simulink model "ControlTest"  (R2016b)
settings: Solver=VariableStepAuto  StartTime=0.0  StopTime=300  MaxStep=0.05  RelTol=1e-3
values from neighbouring files (symbols this model uses):
  X0 = P.x0    [gps.m]
undefined symbols (not defined in the file or in its folder): A, B, C, D, deltaChi, drawplane, GetPosition, P
libraries: simulink x9
settings Model: Creator=CFRPG  LastModifiedBy=CFRPG
settings SolverCC: ZeroCrossAlgorithm=Adaptive

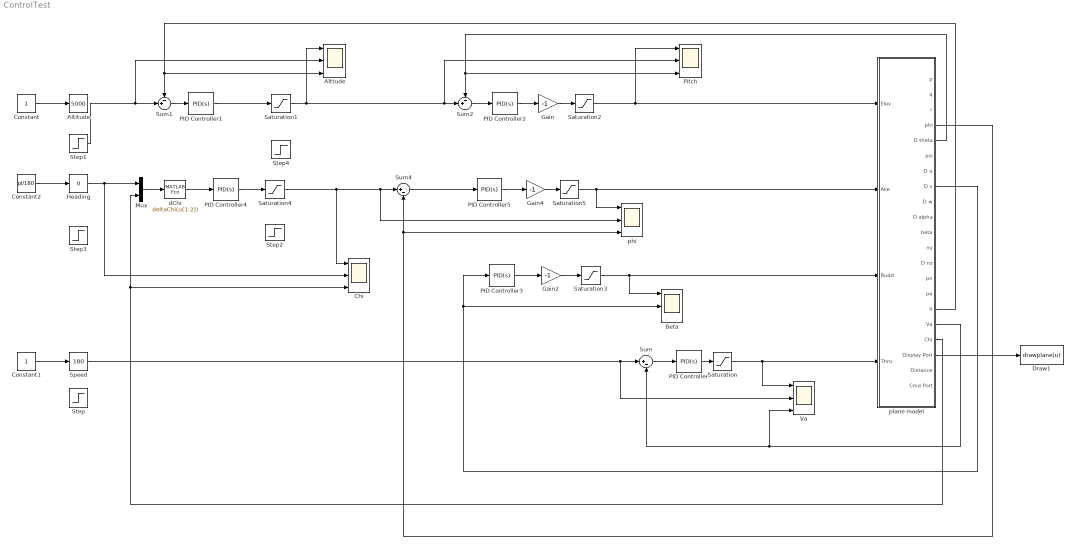
== system ControlTest ==
  Altitude : simulink/Math Operations/Slider Gain  low=0  gain=5000  high=8000
  Alttude : Scope  NumInputPorts=3
  Beta : Scope  NumInputPorts=3
  Chi : Scope  NumInputPorts=3
  Constant : Constant
  Constant1 : Constant
  Constant2 : Constant  Value=pi/180
  Draw1 : MATLABFcn  MATLABFcn=drawplane(u)  OutputDimensions=0
  Gain : Gain  Gain=-1
  Gain2 : Gain  Gain=-1
  Gain4 : Gain  Gain=-1
  Heading : simulink/Math Operations/Slider Gain  low=0  gain=0  high=360
  Mux : Mux  Inputs=2
  PID Controller : simulink/Continuous/PID Controller  Controller=PID  TimeDomain=Continuous-time  SampleTime=-1  IntegratorMethod=Forward Euler  FilterMethod=Forward Euler  Form=Parallel  UseFilter=on  ControllerParametersSource=internal  P=1.6  I=0.001  D=0.01  N=100  InitialConditionSource=internal  InitialConditionForIntegrator=0  InitialConditionForFilter=0  ExternalReset=none  LimitOutput=off  UpperSaturationLimit=inf  LowerSaturationLimit=-inf  LinearizeAsGain=on  AntiWindupMode=none  Kb=1  TrackingMode=off  Kt=1  PParamMin=[]  PParamMax=[]  IParamMin=[]  IParamMax=[]  DParamMin=[]  DParamMax=[]  NParamMin=[]  NParamMax=[]  KbParamMin=[]  KbParamMax=[]  KtParamMin=[]  KtParamMax=[]  POutMin=[]  POutMax=[]  IOutMin=[]  IOutMax=[]  DOutMin=[]  DOutMax=[]  NOutMin=[]  NOutMax=[]  KbOutMin=[]  KbOutMax=[]  KtOutMin=[]  KtOutMax=[]  IntegratorOutMin=[]  IntegratorOutMax=[]  FilterOutMin=[]  FilterOutMax=[]  SumOutMin=[]  SumOutMax=[]  SumI1OutMin=[]  SumI1OutMax=[]  SumI2OutMin=[]  SumI2OutMax=[]  SumI3OutMin=[]  SumI3OutMax=[]  SumDOutMin=[]  SumDOutMax=[]  SaturationOutMin=[]  SaturationOutMax=[]  IntegratorContinuousStateAttributes=''  IntegratorStateMustResolveToSignalObject=off  IntegratorRTWStateStorageClass=Auto  FilterContinuousStateAttributes=''  FilterStateMustResolveToSignalObject=off  FilterRTWStateStorageClass=Auto  DifferentiatorICPrevScaledInput=0  DifferentiatorOutMin=[]  DifferentiatorOutMax=[]
  PID Controller1 : simulink/Continuous/PID Controller  Controller=PID  TimeDomain=Continuous-time  SampleTime=-1  IntegratorMethod=Forward Euler  FilterMethod=Forward Euler  Form=Parallel  UseFilter=on  ControllerParametersSource=internal  P=0.02  I=0.0001  D=0.03  N=100  InitialConditionSource=internal  InitialConditionForIntegrator=0  InitialConditionForFilter=0  ExternalReset=none  LimitOutput=off  UpperSaturationLimit=inf  LowerSaturationLimit=-inf  LinearizeAsGain=on  AntiWindupMode=none  Kb=1  TrackingMode=off  Kt=1  PParamMin=[]  PParamMax=[]  IParamMin=[]  IParamMax=[]  DParamMin=[]  DParamMax=[]  NParamMin=[]  NParamMax=[]  KbParamMin=[]  KbParamMax=[]  KtParamMin=[]  KtParamMax=[]  POutMin=[]  POutMax=[]  IOutMin=[]  IOutMax=[]  DOutMin=[]  DOutMax=[]  NOutMin=[]  NOutMax=[]  KbOutMin=[]  KbOutMax=[]  KtOutMin=[]  KtOutMax=[]  IntegratorOutMin=[]  IntegratorOutMax=[]  FilterOutMin=[]  FilterOutMax=[]  SumOutMin=[]  SumOutMax=[]  SumI1OutMin=[]  SumI1OutMax=[]  SumI2OutMin=[]  SumI2OutMax=[]  SumI3OutMin=[]  SumI3OutMax=[]  SumDOutMin=[]  SumDOutMax=[]  SaturationOutMin=[]  SaturationOutMax=[]  IntegratorContinuousStateAttributes=''  IntegratorStateMustResolveToSignalObject=off  IntegratorRTWStateStorageClass=Auto  FilterContinuousStateAttributes=''  FilterStateMustResolveToSignalObject=off  FilterRTWStateStorageClass=Auto  DifferentiatorICPrevScaledInput=0  DifferentiatorOutMin=[]  DifferentiatorOutMax=[]
  PID Controller2 : simulink/Continuous/PID Controller  Controller=PID  TimeDomain=Continuous-time  SampleTime=-1  IntegratorMethod=Forward Euler  FilterMethod=Forward Euler  Form=Parallel  UseFilter=on  ControllerParametersSource=internal  P=2  I=0.1  D=0.4  N=100  InitialConditionSource=internal  InitialConditionForIntegrator=0  InitialConditionForFilter=0  ExternalReset=none  LimitOutput=off  UpperSaturationLimit=inf  LowerSaturationLimit=-inf  LinearizeAsGain=on  AntiWindupMode=none  Kb=1  TrackingMode=off  Kt=1  PParamMin=[]  PParamMax=[]  IParamMin=[]  IParamMax=[]  DParamMin=[]  DParamMax=[]  NParamMin=[]  NParamMax=[]  KbParamMin=[]  KbParamMax=[]  KtParamMin=[]  KtParamMax=[]  POutMin=[]  POutMax=[]  IOutMin=[]  IOutMax=[]  DOutMin=[]  DOutMax=[]  NOutMin=[]  NOutMax=[]  KbOutMin=[]  KbOutMax=[]  KtOutMin=[]  KtOutMax=[]  IntegratorOutMin=[]  IntegratorOutMax=[]  FilterOutMin=[]  FilterOutMax=[]  SumOutMin=[]  SumOutMax=[]  SumI1OutMin=[]  SumI1OutMax=[]  SumI2OutMin=[]  SumI2OutMax=[]  SumI3OutMin=[]  SumI3OutMax=[]  SumDOutMin=[]  SumDOutMax=[]  SaturationOutMin=[]  SaturationOutMax=[]  IntegratorContinuousStateAttributes=''  IntegratorStateMustResolveToSignalObject=off  IntegratorRTWStateStorageClass=Auto  FilterContinuousStateAttributes=''  FilterStateMustResolveToSignalObject=off  FilterRTWStateStorageClass=Auto  DifferentiatorICPrevScaledInput=0  DifferentiatorOutMin=[]  DifferentiatorOutMax=[]
  PID Controller3 : simulink/Continuous/PID Controller  Controller=PID  TimeDomain=Continuous-time  SampleTime=-1  IntegratorMethod=Forward Euler  FilterMethod=Forward Euler  Form=Parallel  UseFilter=on  ControllerParametersSource=internal  P=0.01  I=0  D=0.01  N=100  InitialConditionSource=internal  InitialConditionForIntegrator=0  InitialConditionForFilter=0  ExternalReset=none  LimitOutput=off  UpperSaturationLimit=inf  LowerSaturationLimit=-inf  LinearizeAsGain=on  AntiWindupMode=none  Kb=1  TrackingMode=off  Kt=1  PParamMin=[]  PParamMax=[]  IParamMin=[]  IParamMax=[]  DParamMin=[]  DParamMax=[]  NParamMin=[]  NParamMax=[]  KbParamMin=[]  KbParamMax=[]  KtParamMin=[]  KtParamMax=[]  POutMin=[]  POutMax=[]  IOutMin=[]  IOutMax=[]  DOutMin=[]  DOutMax=[]  NOutMin=[]  NOutMax=[]  KbOutMin=[]  KbOutMax=[]  KtOutMin=[]  KtOutMax=[]  IntegratorOutMin=[]  IntegratorOutMax=[]  FilterOutMin=[]  FilterOutMax=[]  SumOutMin=[]  SumOutMax=[]  SumI1OutMin=[]  SumI1OutMax=[]  SumI2OutMin=[]  SumI2OutMax=[]  SumI3OutMin=[]  SumI3OutMax=[]  SumDOutMin=[]  SumDOutMax=[]  SaturationOutMin=[]  SaturationOutMax=[]  IntegratorContinuousStateAttributes=''  IntegratorStateMustResolveToSignalObject=off  IntegratorRTWStateStorageClass=Auto  FilterContinuousStateAttributes=''  FilterStateMustResolveToSignalObject=off  FilterRTWStateStorageClass=Auto  DifferentiatorICPrevScaledInput=0  DifferentiatorOutMin=[]  DifferentiatorOutMax=[]
  PID Controller4 : simulink/Continuous/PID Controller  Controller=PID  TimeDomain=Continuous-time  SampleTime=-1  IntegratorMethod=Forward Euler  FilterMethod=Forward Euler  Form=Parallel  UseFilter=on  ControllerParametersSource=internal  P=1.5  I=0  D=1.2  N=100  InitialConditionSource=internal  InitialConditionForIntegrator=0  InitialConditionForFilter=0  ExternalReset=none  LimitOutput=off  UpperSaturationLimit=inf  LowerSaturationLimit=-inf  LinearizeAsGain=on  AntiWindupMode=none  Kb=1  TrackingMode=off  Kt=1  PParamMin=[]  PParamMax=[]  IParamMin=[]  IParamMax=[]  DParamMin=[]  DParamMax=[]  NParamMin=[]  NParamMax=[]  KbParamMin=[]  KbParamMax=[]  KtParamMin=[]  KtParamMax=[]  POutMin=[]  POutMax=[]  IOutMin=[]  IOutMax=[]  DOutMin=[]  DOutMax=[]  NOutMin=[]  NOutMax=[]  KbOutMin=[]  KbOutMax=[]  KtOutMin=[]  KtOutMax=[]  IntegratorOutMin=[]  IntegratorOutMax=[]  FilterOutMin=[]  FilterOutMax=[]  SumOutMin=[]  SumOutMax=[]  SumI1OutMin=[]  SumI1OutMax=[]  SumI2OutMin=[]  SumI2OutMax=[]  SumI3OutMin=[]  SumI3OutMax=[]  SumDOutMin=[]  SumDOutMax=[]  SaturationOutMin=[]  SaturationOutMax=[]  IntegratorContinuousStateAttributes=''  IntegratorStateMustResolveToSignalObject=off  IntegratorRTWStateStorageClass=Auto  FilterContinuousStateAttributes=''  FilterStateMustResolveToSignalObject=off  FilterRTWStateStorageClass=Auto  DifferentiatorICPrevScaledInput=0  DifferentiatorOutMin=[]  DifferentiatorOutMax=[]
  PID Controller5 : simulink/Continuous/PID Controller  Controller=PID  TimeDomain=Continuous-time  SampleTime=-1  IntegratorMethod=Forward Euler  FilterMethod=Forward Euler  Form=Parallel  UseFilter=on  ControllerParametersSource=internal  P=2  I=0  D=0.1  N=100  InitialConditionSource=internal  InitialConditionForIntegrator=0  InitialConditionForFilter=0  ExternalReset=none  LimitOutput=off  UpperSaturationLimit=inf  LowerSaturationLimit=-inf  LinearizeAsGain=on  AntiWindupMode=none  Kb=1  TrackingMode=off  Kt=1  PParamMin=[]  PParamMax=[]  IParamMin=[]  IParamMax=[]  DParamMin=[]  DParamMax=[]  NParamMin=[]  NParamMax=[]  KbParamMin=[]  KbParamMax=[]  KtParamMin=[]  KtParamMax=[]  POutMin=[]  POutMax=[]  IOutMin=[]  IOutMax=[]  DOutMin=[]  DOutMax=[]  NOutMin=[]  NOutMax=[]  KbOutMin=[]  KbOutMax=[]  KtOutMin=[]  KtOutMax=[]  IntegratorOutMin=[]  IntegratorOutMax=[]  FilterOutMin=[]  FilterOutMax=[]  SumOutMin=[]  SumOutMax=[]  SumI1OutMin=[]  SumI1OutMax=[]  SumI2OutMin=[]  SumI2OutMax=[]  SumI3OutMin=[]  SumI3OutMax=[]  SumDOutMin=[]  SumDOutMax=[]  SaturationOutMin=[]  SaturationOutMax=[]  IntegratorContinuousStateAttributes=''  IntegratorStateMustResolveToSignalObject=off  IntegratorRTWStateStorageClass=Auto  FilterContinuousStateAttributes=''  FilterStateMustResolveToSignalObject=off  FilterRTWStateStorageClass=Auto  DifferentiatorICPrevScaledInput=0  DifferentiatorOutMin=[]  DifferentiatorOutMax=[]
  Pitch : Scope  NumInputPorts=3
  Saturation : Saturate  UpperLimit=3  LowerLimit=-3
  Saturation1 : Saturate  UpperLimit=pi/8  LowerLimit=-pi/8
  Saturation2 : Saturate  UpperLimit=pi/9  LowerLimit=-pi/9
  Saturation3 : Saturate  UpperLimit=pi/9  LowerLimit=-pi/9
  Saturation4 : Saturate  UpperLimit=pi/7  LowerLimit=-pi/7
  Saturation5 : Saturate  UpperLimit=pi/9  LowerLimit=-pi/9
  Speed : simulink/Math Operations/Slider Gain  low=180  gain=180  high=340
  Step : Step  Time=5  Before=180  After=264  SampleTime=0
  Step1 : Step  Time=5  Before=300  After=3000  SampleTime=0
  Step2 : Step  Time=5  After=pi/9  SampleTime=0
  Step3 : Step  Time=5  After=pi  SampleTime=0
  Step4 : Step  Time=5  After=pi/9  SampleTime=0
  Sum : Sum  Inputs=|+-
  Sum1 : Sum  Inputs=-+|
  Sum2 : Sum  Inputs=-+|
  Sum4 : Sum  Inputs=|+-
  Va : Scope  NumInputPorts=3
  dChi : MATLABFcn  MATLABFcn=deltaChi(u(1:2))  OutputDimensions=1
  phi : Scope  NumInputPorts=3
  plane model : Subsystem
  wires:
  Saturation/1 -> plane model/4(Thro), Va/1
  PID Controller/1 -> Saturation/1
  Sum/1 -> PID Controller/1
  plane model/17(Va) -> Va/3, Sum/2
  plane model/16(h) -> Sum1/1, Alttude/3
  Step1/1 -> Alttude/2, Sum1/2
  Sum1/1 -> PID Controller1/1
  Sum2/1 -> PID Controller2/1
  Saturation1/1 -> Pitch/2, Sum2/2, Alttude/1
  plane model/5(D theta) -> Sum2/1, Pitch/3
  PID Controller2/1 -> Gain/1
  Constant/1 -> Altitude/1
  Constant1/1 -> Speed/1
  Gain/1 -> Saturation2/1
  PID Controller1/1 -> Saturation1/1
  Speed/1 -> Va/2, Sum/1
  plane model/8(D v) -> PID Controller3/1, Beta/2
  Saturation2/1 -> Pitch/1, plane model/1(Elev)
  PID Controller3/1 -> Gain2/1
  Saturation3/1 -> Beta/1, plane model/3(Rudd)
  Gain2/1 -> Saturation3/1
  plane model/18(Chi) -> Mux/2, Chi/3
  Constant2/1 -> Heading/1
  Heading/1 -> Chi/2, Mux/1
  dChi/1 -> PID Controller4/1
  PID Controller4/1 -> Saturation4/1
  Saturation4/1 -> Chi/1, Sum4/1, phi/2
  plane model/4(phi) -> Sum4/2, phi/3
  Sum4/1 -> PID Controller5/1
  PID Controller5/1 -> Gain4/1
  Gain4/1 -> Saturation5/1
  Saturation5/1 -> phi/1, plane model/2(Alie)
  Mux/1 -> dChi/1
  plane model/19(Display Port) -> Draw1/1

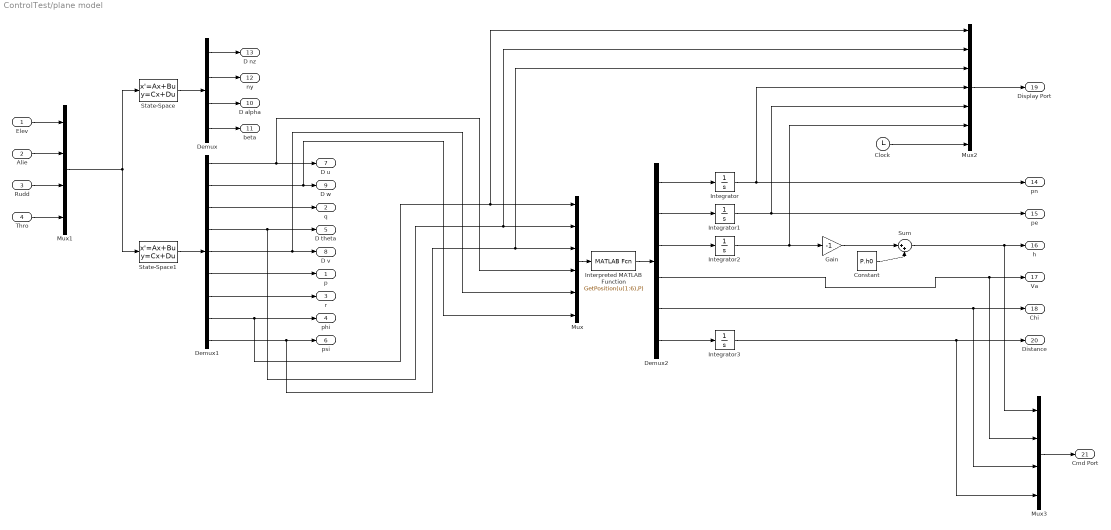
== system ControlTest/plane model ==
  Elev : Inport
  Alie : Inport  Port=2
  Rudd : Inport  Port=3
  Thro : Inport  Port=4
  Clock : Clock
  Constant : Constant  Value=P.h0
  Demux : Demux
  Demux1 : Demux  Outputs=9
  Demux2 : Demux  Outputs=6
  Gain : Gain  Gain=-1
  Integrator{,1..3} (4 alike) : Integrator
  Interpreted MATLAB Function : MATLABFcn  MATLABFcn=GetPosition(u(1:6),P)
  Mux : Mux  Inputs=6
  Mux1 : Mux
  Mux2 : Mux  Inputs=7
  Mux3 : Mux
  State-Space : StateSpace  A=A  B=B  C=C  D=D  X0=X0
  State-Space1 : StateSpace  A=A  B=B  C=eye(9,9)  D=zeros(9,4)  X0=X0
  Sum : Sum  Inputs=|++
  p : Outport
  q : Outport  Port=2
  r : Outport  Port=3
  phi : Outport  Port=4
  D theta : Outport  Port=5
  psi : Outport  Port=6
  D u : Outport  Port=7
  D v : Outport  Port=8
  D w : Outport  Port=9
  D alpha : Outport  Port=10
  beta : Outport  Port=11
  ny : Outport  Port=12
  D nz : Outport  Port=13
  pn : Outport  Port=14
  pe : Outport  Port=15
  h : Outport  Port=16
  Va : Outport  Port=17
  Chi : Outport  Port=18
  Display Port : Outport  Port=19
  Distance : Outport  Port=20
  Cmd Port : Outport  Port=21
  wires:
  Mux1/1 -> State-Space1/1, State-Space/1
  State-Space/1 -> Demux/1
  State-Space1/1 -> Demux1/1
  Demux/1 -> D nz/1
  Demux/2 -> ny/1
  Demux/3 -> D alpha/1
  Demux/4 -> beta/1
  Demux1/2 -> Mux/6, D w/1
  Demux1/1 -> Mux/4, D u/1
  Demux1/3 -> q/1
  Demux1/4 -> D theta/1, Mux2/2, Mux/2
  Demux1/5 -> Mux/5, D v/1
  Demux1/6 -> p/1
  Demux1/7 -> r/1
  Demux1/8 -> Mux2/1, Mux/1, phi/1
  Demux1/9 -> Mux/3, Mux2/3, psi/1
  Mux/1 -> Interpreted MATLAB Function/1
  Interpreted MATLAB Function/1 -> Demux2/1
  Demux2/1 -> Integrator/1
  Demux2/2 -> Integrator1/1
  Demux2/3 -> Integrator2/1
  Integrator/1 -> Mux2/4, pn/1
  Integrator1/1 -> Mux2/5, pe/1
  Gain/1 -> Sum/1
  Integrator2/1 -> Mux2/6, Gain/1
  Demux2/4 -> Mux3/2, Va/1
  Demux2/5 -> Mux3/3, Chi/1
  Elev/1 -> Mux1/1
  Alie/1 -> Mux1/2
  Rudd/1 -> Mux1/3
  Thro/1 -> Mux1/4
  Mux2/1 -> Display Port/1
  Constant/1 -> Sum/2
  Sum/1 -> Mux3/1, h/1
  Clock/1 -> Mux2/7
  Integrator3/1 -> Mux3/4, Distance/1
  Demux2/6 -> Integrator3/1
  Mux3/1 -> Cmd Port/1
